simulink model "V2_Modell_RLC"  (R2021a)
settings: Solver=ode3  StartTime=0.0  StopTime=Zeit(end)  FixedStep=0.000001  RelTol=1e-3
values from neighbouring files (symbols this model uses):
  den = [R_V*C*L*R_d,R_d*L+R_V*L+R_V*R_d*C*R_L,R_V*R_d+R_V*R_L]    [V2_Parameter_RLC_gemessen.m]    (also in V2_Parameter_RLC_nominal.m; V2_Parameter_RLC_optimiert.m)
  num = [R_d*L,R_d*R_L]    [V2_Parameter_RLC_gemessen.m]    (also in V2_Parameter_RLC_nominal.m; V2_Parameter_RLC_optimiert.m)
settings Model: Creator=schmi  LastModifiedBy=schmi

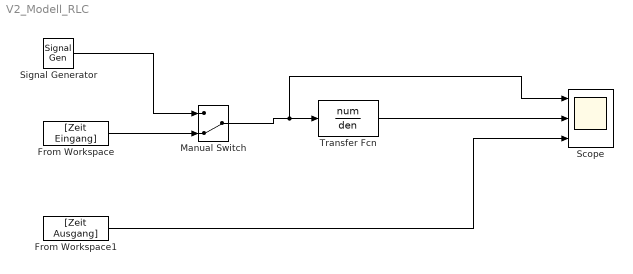
== system V2_Modell_RLC ==
  From Workspace : FromWorkspace  VariableName=[Zeit Eingang]
  From Workspace1 : FromWorkspace  VariableName=[Zeit Ausgang]
  Manual Switch : ManualSwitch  CurrentSetting=0
  Scope : Scope  NumInputPorts=3
  Signal Generator : SignalGenerator  WaveForm=square  Amplitude=-1  Frequency=1000000  Units=rad/sec
  Transfer Fcn : TransferFcn  Numerator=num  Denominator=den
  wires:
  Signal Generator/1 -> Manual Switch/1
  From Workspace/1 -> Manual Switch/2
  Manual Switch/1 -> Scope/1, Transfer Fcn/1
  Transfer Fcn/1 -> Scope/2
  From Workspace1/1 -> Scope/3
